simulink model "simDcControlled"  (R2024a)
settings: Solver=ode45  StartTime=0.0  StopTime=simTimeStop  FixedStep=10^-6  RelTol=1e-3
values from neighbouring files (symbols this model uses):
  Kp = p(1)    [costFunction.m]
undefined symbols (not defined in the file or in its folder): J, Kg, Mgr, Ra, simSaturationHigh, simSaturationLow, simStepAmp, simTimePayload, simValuePayload, Tn
settings Model: Creator=simon  LastModifiedBy=simon
settings SolverCC: EnableFixedStepZeroCrossing=on
settings RTWCC: GPUComputeCapability=3.5

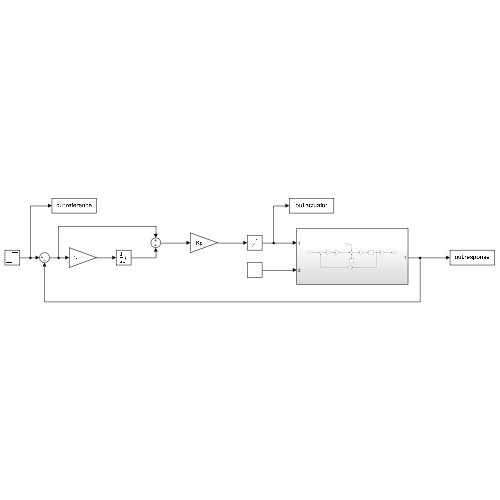
[thumbnail: Simulink's stored preview of the top-level diagram]
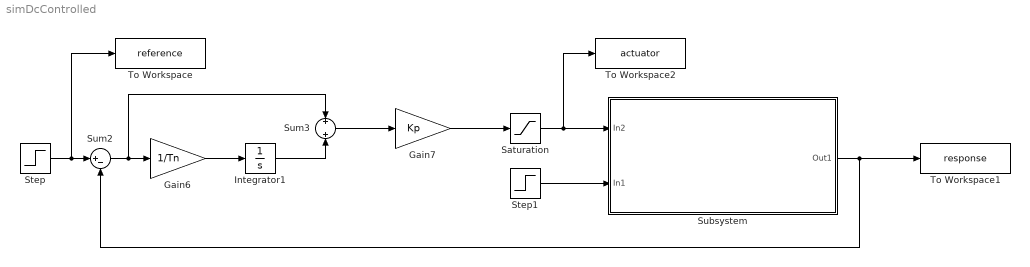
== system simDcControlled ==
  Gain6 : Gain  Gain=1/Tn
  Gain7 : Gain  Gain=Kp
  Integrator1 : Integrator  LimitOutput=on  UpperSaturationLimit=simSaturationHigh  LowerSaturationLimit=simSaturationLow
  Saturation : Saturate  UpperLimit=simSaturationHigh  LowerLimit=simSaturationLow
  Step : Step  Time=0  After=simStepAmp  SampleTime=0
  Step1 : Step  Time=simTimePayload  After=simValuePayload  SampleTime=0
  Subsystem : Subsystem
  Sum2 : Sum  Inputs=|+-
  Sum3 : Sum  Inputs=+||+
  To Workspace : ToWorkspace  VariableName=reference  SaveFormat=Timeseries  SampleTime=-1
  To Workspace1 : ToWorkspace  VariableName=response  SaveFormat=Timeseries  SampleTime=-1
  To Workspace2 : ToWorkspace  VariableName=actuator  SaveFormat=Timeseries  SampleTime=-1
  wires:
  Step/1 -> To Workspace/1, Sum2/1
  Sum2/1 -> Sum3/1, Gain6/1
  Gain6/1 -> Integrator1/1
  Integrator1/1 -> Sum3/2
  Sum3/1 -> Gain7/1
  Gain7/1 -> Saturation/1
  Step1/1 -> Subsystem/2(In1)
  Saturation/1 -> To Workspace2/1, Subsystem/1(In2)
  Subsystem/1(Out1) -> To Workspace1/1, Sum2/2

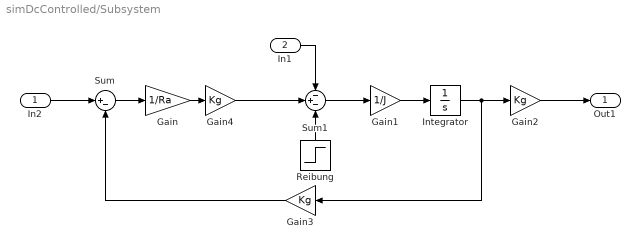
== system simDcControlled/Subsystem ==
  In2 : Inport
  In1 : Inport  Port=2
  Gain : Gain  Gain=1/Ra
  Gain1 : Gain  Gain=1/J
  Gain2 : Gain  Gain=Kg
  Gain3 : Gain  Gain=Kg
  Gain4 : Gain  Gain=Kg
  Integrator : Integrator
  Reibung : Step  Time=0  After=Mgr  SampleTime=0
  Sum : Sum  Inputs=|+-
  Sum1 : Sum  Inputs=-+-
  Out1 : Outport
  wires:
  Reibung/1 -> Sum1/3
  Gain3/1 -> Sum/2
  Integrator/1 -> Gain3/1, Gain2/1
  Gain1/1 -> Integrator/1
  Gain4/1 -> Sum1/2
  Gain/1 -> Gain4/1
  Gain2/1 -> Out1/1
  In2/1 -> Sum/1
  Sum/1 -> Gain/1
  Sum1/1 -> Gain1/1
  In1/1 -> Sum1/1
